simulink model "SRF_PLL"  (R2025a)
settings: Solver=VariableStepAuto  StartTime=0.0  StopTime=0.3  RelTol=1e-3
libraries: slpidlib x1, simulink x1, spsabctodq0Lib x1
settings Model: Creator=lucaslee  LastModifiedBy=lucaslee

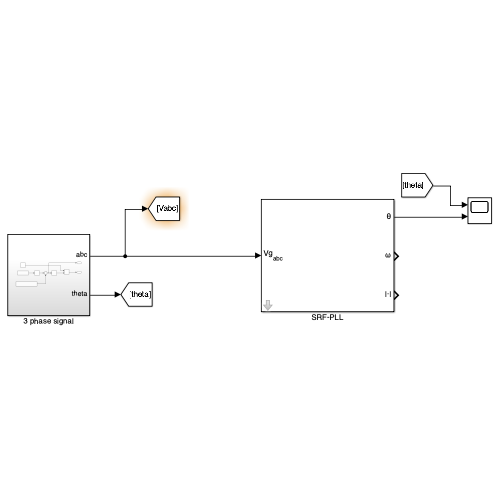
[thumbnail: Simulink's stored preview of the top-level diagram]
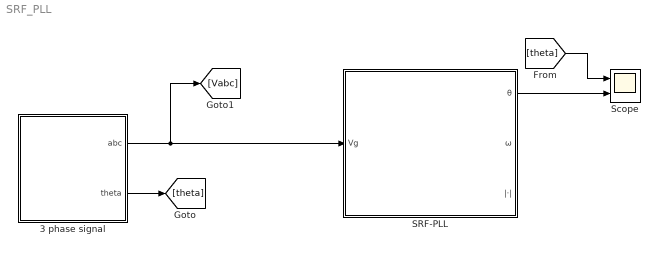
== system SRF_PLL ==
  3 phase signal : Subsystem
  SRF-PLL : Subsystem  mask(DSOGI-PLL){FREQ=50, zeta=1/sqrt(2), BW=30, F_out=on, fc=15}
      mask prompts: FREQ "Nominal frequency [Hz]"; zeta "SRF-PLL Damping factor ζ"; BW "SRF-PLL Bandwidth [Hz]"; F_out "Frequency output filter"; fc "LPF cut off frequency [Hz]"
      mask help:
      | This blocks implements a three-phase PLL based on a second order generalized integrator.
      |
      | Return values are in radian [0.2pi[ for the phase, in rad/s for the frequency and in the same unit as the input for the voltage.
      mask Help: https://imperix.com/doc/implementation/synchronous-reference-frame-pll
      mask DialogControl DescGroupVar Prompt: SRF-PLL
      mask DialogControl DescTextVar Prompt: This blocks implements a three phase synchronous reference frame PLL.
      mask DialogControl Control2 Prompt: Return values are in radian [0.2pi[ for the phase, in rad/s for the frequency and in the same unit as the input for the voltage.
      mask DialogControl Container4 Prompt: Parameters
      mask DialogControl Container5 Prompt: Frequency output
      mask Display:
      | %Print the block type:
      | color('black');
      | port_label('input',1,'Vg_{abc}','texmode','on');
      | port_label('output',1,'\theta','texmode','on');
      | port_label('output',2,'\omega','texmode','on');
      | port_label('output',3,'|·|','texmode','on');
  Scope : Scope  NumInputPorts=2
      settings: ActiveDisplayYMinimum=-17.98238663857272  ActiveDisplayYMaximum=87.035731613577227
  wires:
  3 phase signal/2(theta) -> [theta]
  SRF-PLL/1(θ) -> Scope/2
  [theta] -> Scope/1
  3 phase signal/1(abc) -> SRF-PLL/1(Vg), [Vabc]

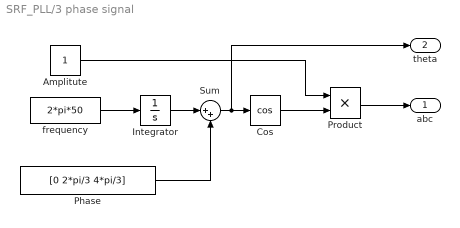
== system SRF_PLL/3 phase signal ==
  Amplitute : Constant
  Cos : Trigonometry  Operator=cos
  Integrator : Integrator
  Phase : Constant  Value=[0 2*pi/3 4*pi/3]
  Product : Product
  Sum : Sum  Inputs=|++
  frequency : Constant  Value=2*pi*50
  abc : Outport
  theta : Outport  Port=2
  wires:
  Product/1 -> abc/1
  frequency/1 -> Integrator/1
  Amplitute/1 -> Product/1
  Integrator/1 -> Sum/1
  Phase/1 -> Sum/2
  Sum/1 -> theta/1, Cos/1
  Cos/1 -> Product/2

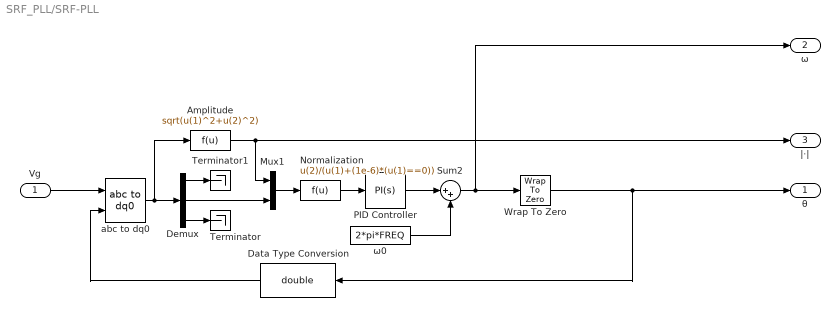
== system SRF_PLL/SRF-PLL ==
  Vg : Inport
  Amplitude : Fcn  Expr=sqrt(u(1)^2+u(2)^2)
  Data Type Conversion : DataTypeConversion  OutDataTypeStr=double  SaturateOnIntegerOverflow=off  RndMeth=Floor
  Demux : Demux  Outputs=3
  Mux1 : Mux  Inputs=2
  Normalization : Fcn  Expr=u(2)/(u(1)+(1e-6)*(u(1)==0))
  PID Controller : slpidlib/PID Controller  Controller=PI  Form=Parallel  TimeDomain=Continuous-time  UseExternalTs=off  SampleTime=-1  IntegratorMethod=Forward Euler  FilterMethod=Forward Euler  ControllerParametersSource=internal  P=2*2*pi*BW*zeta  I=BW*BW*4*pi*pi  UseKiTs=off  D=0  UseExternalDerivativeSource=off  N=100  UseFilter=on  TunerSelectOption=Transfer Function Based (PID Tuner App)  InitialConditionSource=internal  InitialConditionForIntegrator=0  InitialConditionForFilter=0  DifferentiatorICPrevScaledInput=0  ExternalReset=none  TrackingMode=off  Kt=1  LimitOutput=off  SatLimitsSource=internal  UpperSaturationLimit=inf  LowerSaturationLimit=-inf  LinearizeAsGain=on  AntiWindupMode=none  Kb=1  LimitIntegrator=off  UpperIntegratorSaturationLimit=inf  LowerIntegratorSaturationLimit=-inf  POutMin=[]  POutMax=[]  IOutMin=[]  IOutMax=[]  DOutMin=[]  DOutMax=[]  NOutMin=[]  NOutMax=[]  SumOutMin=[]  SumOutMax=[]  SaturationOutMin=[]  SaturationOutMax=[]  PParamMin=[]  PParamMax=[]  IParamMin=[]  IParamMax=[]  DParamMin=[]  DParamMax=[]  NParamMin=[]  NParamMax=[]  KbParamMin=[]  KbParamMax=[]  KtParamMin=[]  KtParamMax=[]  KbOutMin=[]  KbOutMax=[]  KtOutMin=[]  KtOutMax=[]  IntegratorOutMin=[]  IntegratorOutMax=[]  FilterOutMin=[]  FilterOutMax=[]  SumI1OutMin=[]  SumI1OutMax=[]  SumI2OutMin=[]  SumI2OutMax=[]  SumI3OutMin=[]  SumI3OutMax=[]  SumI4OutMin=[]  SumI4OutMax=[]  SumDOutMin=[]  SumDOutMax=[]  DifferentiatorOutMin=[]  DifferentiatorOutMax=[]  FilterDiffOutCoefMin=[]  FilterDiffOutCoefMax=[]  ReciprocalOutMin=[]  ReciprocalOutMax=[]  SumDenOutMin=[]  SumDenOutMax=[]  SumNumOutMin=[]  SumNumOutMax=[]  DivideOutMin=[]  DivideOutMax=[]  UdiffTsProdOutMin=[]  UdiffTsProdOutMax=[]  NTsProdOutMin=[]  NTsProdOutMax=[]  UintegralTsProdOutMin=[]  UintegralTsProdOutMax=[]  UngainTsProdOutMin=[]  UngainTsProdOutMax=[]  ClampingZeroOutDataTypeStr=Inherit: Inherit via back propagation  ClampingZeroOutMin=[]  ClampingZeroOutMax=[]  FilterDenConstantOutDataTypeStr=Inherit: Inherit via back propagation  FilterDenConstantOutMin=[]  FilterDenConstantOutMax=[]  PCopyOutDataTypeStr=Inherit: Inherit via back propagation  PCopyOutMin=[]  PCopyOutMax=[]  NCopyOutDataTypeStr=Inherit: Inherit via back propagation  NCopyOutMin=[]  NCopyOutMax=[]  IntegratorContinuousStateAttributes=''  IntegratorStateMustResolveToSignalObject=off  IntegratorRTWStateStorageClass=Auto  FilterContinuousStateAttributes=''  FilterStateMustResolveToSignalObject=off  FilterRTWStateStorageClass=Auto  ParallelPVariant=InternalParameters  IdealPVariant=Disabled  IVariant=InternalParameters  DVariant=Disabled  IntegratorVariant=Continuous  SatVariant=Disabled  AWVariant=Passthrough  PCopyVariant=Disabled  TRVariant=Disabled  FdbkBlocksVariant=Forward  IdealPFdbkVariant=Disabled  SatFdbkVariant=Disabled  DerivativeFilterVariant=Disabled  NVariant=Disabled  NCopyVariant=Disabled_SignalSpec  FilterICVariant=Disabled  IntegratorICVariant=InternalICs  ExternalResetVariant=Disabled  TRSumVariant=Passthrough  SumFdbkVariant=Disabled  SumVariant=Sum_PI  TsampFilterVariant=InternalTs  TsampNgainVariant=Passthrough  TsampIntegralVariant=Disabled_SignalSpec  ExternalSaturationOutDataTypeStr=Inherit: Same as second input  DerivativeSourceVariant=Disabled  PreIntVariant=InternalPreInt
  Sum2 : Sum  Inputs=|++
  Terminator : Terminator
  Terminator1 : Terminator
  Wrap To Zero : simulink/Discontinuities/Wrap To Zero  Threshold=2*pi
  abc to dq0 : spsabctodq0Lib/abc to dq0  Alignment=90 degrees behind phase A axis
  ω0 : Constant  Value=2*pi*FREQ  OutDataTypeStr=single
  θ : Outport  OutDataTypeStr=single
  ω : Outport  Port=2  OutDataTypeStr=single
  |·| : Outport  Port=3  OutDataTypeStr=single
  wires:
  ω0/1 -> Sum2/2
  abc to dq0/1 -> Demux/1, Amplitude/1
  Amplitude/1 -> Mux1/1, |·|/1
  Mux1/1 -> Normalization/1
  Wrap To Zero/1 -> Data Type Conversion/1, θ/1
  Normalization/1 -> PID Controller/1
  PID Controller/1 -> Sum2/1
  Vg/1 -> abc to dq0/1
  Sum2/1 -> ω/1, Wrap To Zero/1
  Demux/3 -> Terminator/1
  Demux/1 -> Terminator1/1
  Demux/2 -> Mux1/2
  Data Type Conversion/1 -> abc to dq0/2
